simulink model "L0601d"  (Simulink 10.2)
settings: Solver=VariableStepDiscrete  StartTime=0.0  StopTime=inf  MaxStep=0.1  RelTol=1e-3
settings Model: Creator=Ranci  LastModifiedBy=Ranci
settings DataIOCC: SaveFormat=Dataset  SignalLoggingSaveFormat=Dataset  ReturnWorkspaceOutputs=on
settings OptimizationCC: LifeSpan=auto
settings DebuggingCC: UnderspecifiedInitializationDetection=Simplified  MergeDetectMultiDrivingBlocksExec=error  FcnCallInpInsideContextMsg=error  SFUnexpectedBacktrackingDiag=error  SFNoUnconditionalDefaultTransitionDiag=error  SFExecutionAtInitializationDiag=warning  ArithmeticOperatorsInVariantConditions=error
settings HardwareCC: ProdBitPerPointer=64  ProdBitPerSizeT=64  ProdBitPerPtrDiffT=64  ProdLargestAtomicFloat=Float  ProdIntDivRoundTo=Zero  ProdEndianess=LittleEndian  ProdWordSize=64  ProdHWDeviceType=Intel->x86-64 (Windows64)
settings ModelReferenceCC: PropagateSignalLabelsOutOfModel=on
settings SFSimCC: SimUseLocalCustomCode=on  CustomCodeUndefinedFunction=FilterOut
settings RTWCC: RTWUseLocalCustomCode=on
settings CodeAppCC: StateflowObjectComments=off
settings GRTTargetCC: TargetLangStandard=C99 (ISO)  CombineOutputUpdateFcns=on  GRTInterface=off
settings ConfigComp: CovMetricSettings=dwe  CovSaveCumulativeToWorkspaceVar=off  CovSaveSingleToWorkspaceVar=off  CovExternalEMLEnable=on

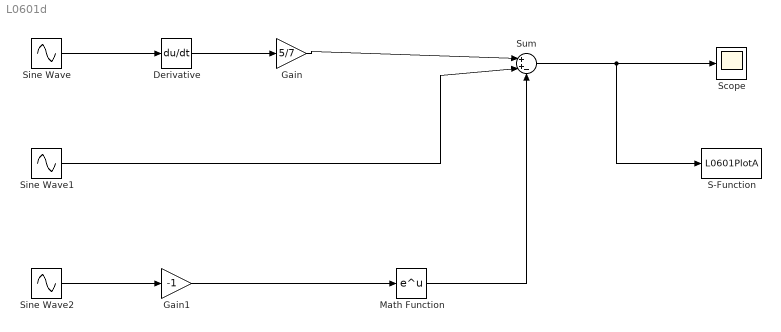
== system L0601d ==
  Derivative : Derivative
  Gain : Gain  Gain=5/7
  Gain1 : Gain  Gain=-1
  Math Function : Math  SaturateOnIntegerOverflow=on
  S-Function : S-Function  FunctionName=L0601PlotA  Parameters=0.1  SFunctionDeploymentMode=off  EnableBusSupport=off
  Scope : Scope
  Sine Wave : Sin  Frequency=7  Phase=pi/2  SampleTime=0
  Sine Wave1 : Sin  Frequency=5  SampleTime=0
  Sine Wave2 : Sin  Frequency=23  SampleTime=0
  Sum : Sum  Inputs=|++-
  wires:
  Sine Wave/1 -> Derivative/1
  Derivative/1 -> Gain/1
  Gain/1 -> Sum/1
  Sine Wave1/1 -> Sum/2
  Sine Wave2/1 -> Gain1/1
  Gain1/1 -> Math Function/1
  Math Function/1 -> Sum/3
  Sum/1 -> S-Function/1, Scope/1
